simulink model "THERM_FMU_MR"  (R2025b)
settings: Solver=FixedStepAuto  StartTime=0.0  StopTime=20  RelTol=1e-3
values from neighbouring files (symbols this model uses):
  TsELEC = 5e-05    [initParams.mat]
settings Model: Creator=gdudgeon  LastModifiedBy=gdudgeon
settings SolverCC: AlgebraicLoopSolver=TrustRegion
settings DebuggingCC: UnconnectedInputMsg=warning  UnconnectedOutputMsg=warning  UnconnectedLineMsg=warning
settings ModelReferenceCC: EnableRefExpFcnMdlSchedulingChecks=on
settings RTWCC: GPUComputeCapability=3.5

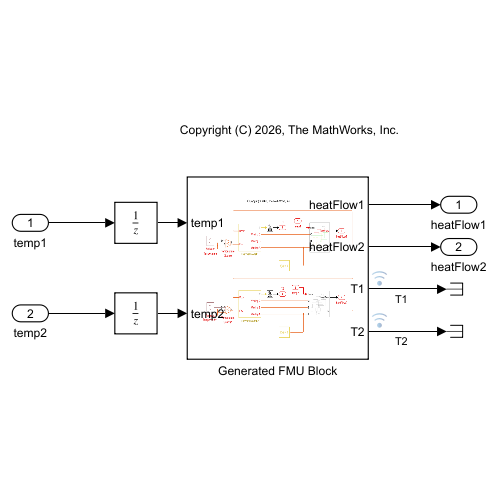
[thumbnail: Simulink's stored preview of the top-level diagram]
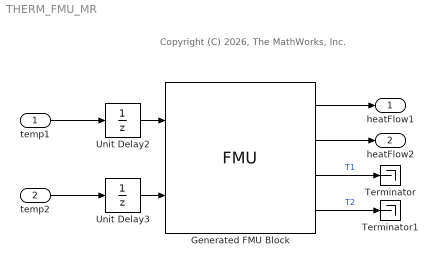
== system THERM_FMU_MR ==
  note: Copyright (C) 2026, The MathWorks, Inc.
  temp1 : Inport  PortDimensions=4  SampleTime=TsELEC
  temp2 : Inport  Port=2  PortDimensions=4  SampleTime=TsELEC
  Generated FMU Block : FMU  FMUName=THERM_FMU  FMUMode=CoSimulation  FMUSampleTime=TsELEC  FMUCreateBusObject=off
      mask Type: THERM_FMU [Co-Simulation, v2.0]
      mask Display:
      | if (exist([Simulink.fileGenControl('get','CacheFolder') '\slprj\_fmu\3e4246507cdc4f8dc3bdcdd2d3f7a88a\THERM_FMU\model.png'],'file'))
      |     image([Simulink.fileGenControl('get','CacheFolder') '\slprj\_fmu\3e4246507cdc4f8dc3bdcdd2d3f7a88a\THERM_FMU\model.png']);
      | else
      |     disp('THERM_FMU');
      | end
      | port_label('output',1,'heatFlow1');
      | port_label('output',2,'heatFlow2');
      | port_label('output',3,'T1');
      | port_label('output',4,'T2');
      | port_label('input',1,'temp1');
      | port_label('input',2,'temp2');
  Terminator : Terminator
  Terminator1 : Terminator
  Unit Delay2 : UnitDelay  SampleTime=-1  HasFrameUpgradeWarning=on
  Unit Delay3 : UnitDelay  SampleTime=-1  HasFrameUpgradeWarning=on
  heatFlow1 : Outport  SampleTime=TsELEC
  heatFlow2 : Outport  Port=2  SampleTime=TsELEC
  wires:
  Generated FMU Block/4 -> Terminator1/1  "T2"
  Generated FMU Block/3 -> Terminator/1  "T1"
  temp1/1 -> Unit Delay2/1
  temp2/1 -> Unit Delay3/1
  Generated FMU Block/1 -> heatFlow1/1
  Generated FMU Block/2 -> heatFlow2/1
  Unit Delay2/1 -> Generated FMU Block/1
  Unit Delay3/1 -> Generated FMU Block/2
